simulink model "starmac_system_minimal"  (Simulink 7.1)
settings: Solver=ode45  StartTime=0.0  StopTime=30  FixedStep=.001  MaxStep=.01  RelTol=1e-4
settings Model: Creator=Administrator  LastModifiedBy=Administrator

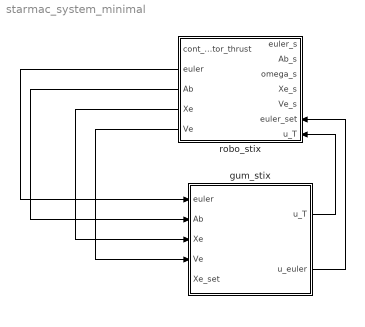
== system starmac_system_minimal ==
  gum_stix : Subsystem
  robo_stix : Subsystem  Orientation=left
  wires:
  robo_stix/2(euler) -> gum_stix/1(euler)
  robo_stix/4(Xe) -> gum_stix/3(Xe)
  robo_stix/5(Ve) -> gum_stix/4(Ve)
  gum_stix/1(u_T) -> robo_stix/7(u_T)
  gum_stix/2(u_euler) -> robo_stix/6(euler_set)
  robo_stix/3(Ab) -> gum_stix/2(Ab)

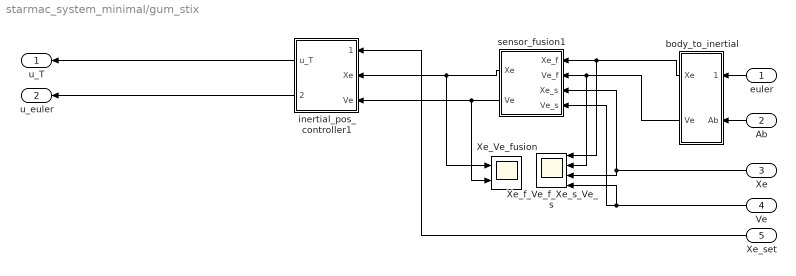
== system starmac_system_minimal/gum_stix ==
  euler : Inport  Orientation=left  PortDimensions=3  DataType=single  OutDataTypeStr=single
  Ab : Inport  Orientation=left  Port=2  PortDimensions=3  DataType=single  OutDataTypeStr=single
  Xe : Inport  Orientation=left  Port=3  PortDimensions=3  DataType=single  OutDataTypeStr=single
  Ve : Inport  Orientation=left  Port=4  PortDimensions=3  DataType=single  OutDataTypeStr=single
  Xe_set : Inport  Orientation=left  Port=5  PortDimensions=3  DataType=single  OutDataTypeStr=single
  Xe_Ve_fusion : Scope  NumInputPorts=2
      settings: YMin=-10~-5  YMax=10~5  SaveName=ScopeData2
  Xe_f_Ve_f_Xe_s_Ve_s : Scope  NumInputPorts=4
      settings: YMin=-5~-5~-5~-5  YMax=5~5~5~5  SaveName=ScopeData3
  body_to_inertial : Subsystem  Orientation=left
  inertial_pos_controller1 : Subsystem  Orientation=left
  sensor_fusion1 : Subsystem  Orientation=left
  u_T : Outport  Orientation=left  PortDimensions=1  DataType=single  OutDataTypeStr=single
  u_euler : Outport  Orientation=left  Port=2  PortDimensions=3  DataType=single  OutDataTypeStr=single
  wires:
  Xe_set/1 -> inertial_pos_controller1/1(Xe_set)
  inertial_pos_controller1/1(u_T) -> u_T/1
  inertial_pos_controller1/2(u_euler) -> u_euler/1
  euler/1 -> body_to_inertial/1(euler)
  Ab/1 -> body_to_inertial/2(Ab)
  sensor_fusion1/1(Xe) -> Xe_Ve_fusion/1, inertial_pos_controller1/2(Xe)
  sensor_fusion1/2(Ve) -> Xe_Ve_fusion/2, inertial_pos_controller1/3(Ve)
  body_to_inertial/1(Xe) -> Xe_f_Ve_f_Xe_s_Ve_s/1, sensor_fusion1/1(Xe_f)
  body_to_inertial/2(Ve) -> Xe_f_Ve_f_Xe_s_Ve_s/2, sensor_fusion1/2(Ve_f)
  Xe/1 -> Xe_f_Ve_f_Xe_s_Ve_s/3, sensor_fusion1/3(Xe_s)
  Ve/1 -> Xe_f_Ve_f_Xe_s_Ve_s/4, sensor_fusion1/4(Ve_s)

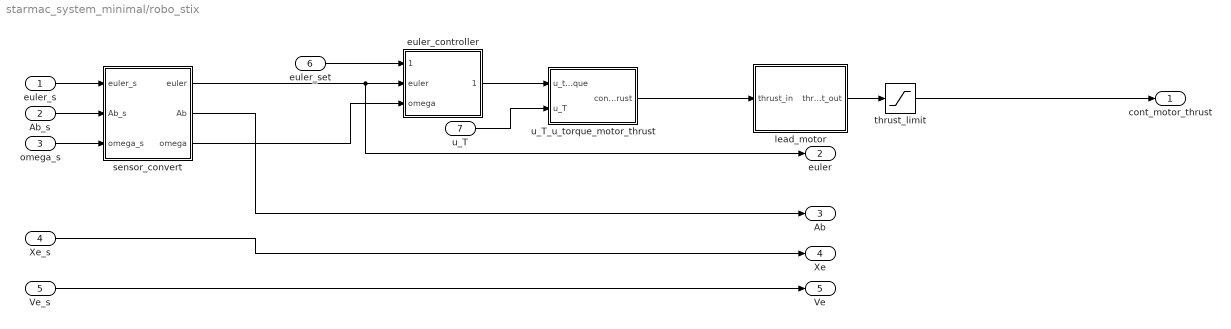
== system starmac_system_minimal/robo_stix ==
  euler_s : Inport  PortDimensions=3  DataType=single  OutDataTypeStr=single
  Ab_s : Inport  Port=2  PortDimensions=3  DataType=single  OutDataTypeStr=single
  omega_s : Inport  Port=3  PortDimensions=3  DataType=single  OutDataTypeStr=single
  Xe_s : Inport  Port=4  PortDimensions=3  DataType=single  OutDataTypeStr=single
  Ve_s : Inport  Port=5  PortDimensions=3  DataType=single  OutDataTypeStr=single
  euler_set : Inport  Port=6  PortDimensions=3  DataType=single  OutDataTypeStr=single
  u_T : Inport  Port=7  PortDimensions=1  DataType=single  OutDataTypeStr=single
  euler_controller : Subsystem  mask{K=1, K_e=7.5, K_o=.65}
      mask prompts: K "Loop Gain [K]:"; K_e "Euler Gain [K_e]:"; K_o "Omega Gain [K_o]:"
  lead_motor : Subsystem  mask{tau_motor=.10, t_s=.020}
      mask init:
      | a=1/tau_motor;
      | b=pi/t_s;
      | T=t_s;
      | num1=b*(1-exp(-b*T))+a*(b*T-1+exp(-b*T));
      | num2=-b*(1-exp(-b*T))+a*(1-exp(-b*T)-b*T*exp(-b*T));
      | den1=a*b;
      | den2=-a*b*exp(-b*T);
      | num=[num1 num2];
      | den=[den1 den2];
      | Hz=tf(num,den,T);
      | [y,t]=step(Hz);
      | k_ss=(1/y(length(y)));
      | num=k_ss*num;
      | lead_a_1=single(-den(2)/den(1))
      | lead_b_1=single(num(2)/den(1))
      | lead_b_2=single(num(1)/den(1))
      | %Hz=k_ss*Hz
      | %bode(Hz);
  sensor_convert : Subsystem  mask{a_g_s=7000, g_g_s=8500}
      mask prompts: a_g_s "AccelGainScale[a_g_s]:"; g_g_s "GyroGainScale[g_g_s]:"
  thrust_limit : Saturate  UpperLimit=10*ones(1,4)  LowerLimit=0*ones(1,4)  OutDataTypeMode=single  OutDataType=sfix(16)  OutScaling=2^0  OutDataTypeStr=single
  u_T_u_torque_motor_thrust : Subsystem  mask{dx=.3048, K_torque=.47}
      mask prompts: dx "X distance of motor from CG [dx](meters):"; K_torque "Ktorque [K_torque]:"
      mask init:
      | M=[0 -dx 0 dx;
      |    dx 0 -dx 0;
      |    -K_torque K_torque -K_torque K_torque;
      |    1 1 1 1];
      | Mi=inv(M);
  cont_motor_thrust : Outport  PortDimensions=4  DataType=single  OutDataTypeStr=single
  euler : Outport  Port=2
  Ab : Outport  Port=3
  Xe : Outport  Port=4
  Ve : Outport  Port=5
  wires:
  euler_s/1 -> sensor_convert/1(euler_s)
  Ab_s/1 -> sensor_convert/2(Ab_s)
  omega_s/1 -> sensor_convert/3(omega_s)
  sensor_convert/1(euler) -> euler/1, euler_controller/2(euler)
  euler_set/1 -> euler_controller/1(euler_set)
  sensor_convert/3(omega) -> euler_controller/3(omega)
  u_T/1 -> u_T_u_torque_motor_thrust/2(u_T)
  Xe_s/1 -> Xe/1
  Ve_s/1 -> Ve/1
  euler_controller/1(u_torque) -> u_T_u_torque_motor_thrust/1(u_torque)
  sensor_convert/2(Ab) -> Ab/1
  u_T_u_torque_motor_thrust/1(cont_motor_thrust) -> lead_motor/1(thrust_in)
  thrust_limit/1 -> cont_motor_thrust/1
  lead_motor/1(thrust_out) -> thrust_limit/1

== system starmac_system_minimal/gum_stix/body_to_inertial ==
  euler : Inport  DataType=single  OutDataTypeStr=single
  Ab : Inport  Port=2  DataType=single  OutDataTypeStr=single
  Ab_to_Ae : Stateflow chart
  inertial_vel_and pos_est : Subsystem  mask{Ts=.02}
      mask prompts: Ts "Sample Time [Ts] (seconds):"
  Xe : Outport
  Ve : Outport  Port=2
  wires:
  inertial_vel_and pos_est/2(Xb) -> Xe/1
  inertial_vel_and pos_est/1(Vb) -> Ve/1
  Ab_to_Ae/1(Ae) -> inertial_vel_and pos_est/1(Ab)
  Ab/1 -> Ab_to_Ae/2(Ab)
  euler/1 -> Ab_to_Ae/1(euler)

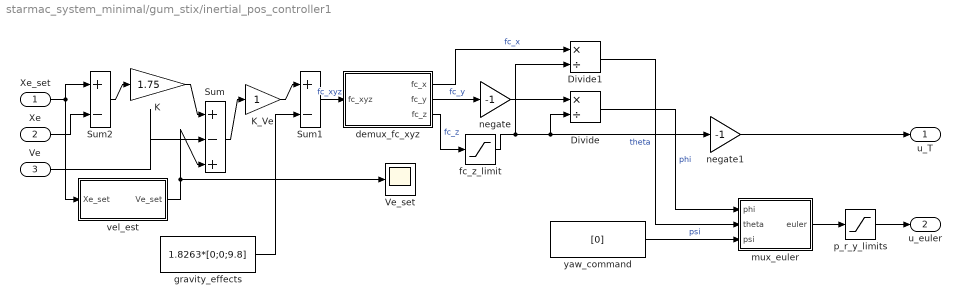
== system starmac_system_minimal/gum_stix/inertial_pos_controller1 ==
  Xe_set : Inport
  Xe : Inport  Port=2
  Ve : Inport  Port=3
  Divide : Product  Inputs=*/  OutDataTypeMode=single  OutDataType=sfix(16)  OutScaling=2^-10  OutDataTypeStr=single
  Divide1 : Product  Inputs=*/  OutDataTypeMode=single  OutDataType=sfix(16)  OutScaling=2^-10  OutDataTypeStr=single
  K : Gain  Gain=1.75  ParameterDataTypeMode=single  ParameterDataType=sfix(16)  ParameterScaling=2^0  ParamDataTypeStr=single  OutDataTypeMode=single  OutDataType=sfix(16)  OutScaling=2^0  OutDataTypeStr=single
  K_Ve : Gain  ParameterDataTypeMode=single  ParameterDataType=sfix(16)  ParameterScaling=2^0  ParamDataTypeStr=single  OutDataTypeMode=single  OutDataType=sfix(16)  OutScaling=2^0  OutDataTypeStr=single
  Sum : Sum  Inputs=|+-+  AccumDataTypeStr=single  OutDataTypeMode=single  OutDataType=sfix(16)  OutScaling=2^0  OutDataTypeStr=single
  Sum1 : Sum  Inputs=|+-  AccumDataTypeStr=single  OutDataTypeMode=single  OutDataType=sfix(16)  OutScaling=2^0  OutDataTypeStr=single
  Sum2 : Sum  Inputs=|+-  AccumDataTypeStr=single  OutDataTypeMode=single  OutDataType=sfix(16)  OutScaling=2^0  OutDataTypeStr=single
  Ve_set : Scope
      settings: SaveName=ScopeData2  Decimation=10
  demux_fc_xyz : Stateflow chart
  fc_z_limit : Saturate  UpperLimit=-(1/4)*9.81  LowerLimit=-4*9.81  OutDataTypeMode=single  OutDataType=sfix(16)  OutScaling=2^0  OutDataTypeStr=single
  gravity_effects : Constant  Value=1.8263*[0;0;9.8]  OutDataTypeMode=single  OutDataType=sfix(16)  OutScaling=2^0  OutDataTypeStr=single
  mux_euler : Stateflow chart
  negate : Gain  Gain=-1  ParameterDataTypeMode=single  ParameterDataType=sfix(16)  ParameterScaling=2^0  ParamDataTypeStr=single  OutDataTypeMode=single  OutDataType=sfix(16)  OutScaling=2^0  OutDataTypeStr=single
  negate1 : Gain  Gain=-1  ParameterDataTypeMode=single  ParameterDataType=sfix(16)  ParameterScaling=2^0  ParamDataTypeStr=single  OutDataTypeMode=single  OutDataType=sfix(16)  OutScaling=2^0  OutDataTypeStr=single
  p_r_y_limits : Saturate  UpperLimit=(pi/4)*ones(1,3)  LowerLimit=-(pi/4)*ones(1,3)  OutDataTypeMode=single  OutDataType=sfix(16)  OutScaling=2^0  OutDataTypeStr=single
  vel_est : Subsystem  mask{tau_f=.02/pi, T=.02}
      mask prompts: T "sample rate"
      mask init:
      | b=1/tau_f;
      | num1=(1-exp(-b*T));
      | num2=-num1;
      | den1=1;
      | den2=-exp(-b*T);
      | num=(1/T)*[num1 num2];
      | den=[den1 den2];
      | vel_est_a_1=single(-den(2)/den(1))
      | vel_est_b_1=single(num(2)/den(1))
      | vel_est_b_2=single(num(1)/den(1))
      | %Hz=tf(num,den,T);
      | %bode(Hz);
      | %hold on;
      | %bode(tf([1 0],[tau_f 1]));
  yaw_command : Constant  Value=[0]  OutDataTypeMode=single  OutDataType=sfix(16)  OutScaling=2^0  OutDataTypeStr=single
  u_T : Outport  DataType=single  OutDataTypeStr=single
  u_euler : Outport  Port=2  PortDimensions=[3]  DataType=single  OutDataTypeStr=single
  wires:
  vel_est/1(Ve_set) -> Ve_set/1, Sum/3
  Ve/1 -> Sum/2
  K_Ve/1 -> Sum1/1
  demux_fc_xyz/2(fc_y) -> negate/1  "fc_y"
  K/1 -> Sum/1
  Sum2/1 -> K/1
  Xe/1 -> Sum2/2
  Sum/1 -> K_Ve/1
  gravity_effects/1 -> Sum1/2
  Sum1/1 -> demux_fc_xyz/1(fc_xyz)  "fc_xyz"
  mux_euler/1(euler) -> p_r_y_limits/1
  demux_fc_xyz/3(fc_z) -> fc_z_limit/1  "fc_z"
  yaw_command/1 -> mux_euler/3(psi)  "psi"
  negate/1 -> Divide/1
  Divide/1 -> mux_euler/1(phi)  "phi"
  demux_fc_xyz/1(fc_x) -> Divide1/1  "fc_x"
  Divide1/1 -> mux_euler/2(theta)  "theta"
  p_r_y_limits/1 -> u_euler/1
  negate1/1 -> u_T/1
  Xe_set/1 -> vel_est/1(Xe_set), Sum2/1
  fc_z_limit/1 -> negate1/1, Divide/2, Divide1/2

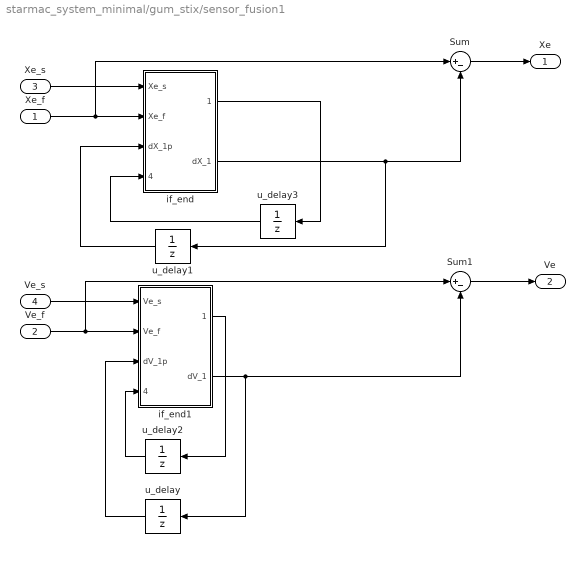
== system starmac_system_minimal/gum_stix/sensor_fusion1 ==
  Xe_f : Inport
  Ve_f : Inport  Port=2
  Xe_s : Inport  Port=3
  Ve_s : Inport  Port=4
  Sum : Sum  Inputs=|+-  OutDataTypeMode=single  OutDataType=sfix(16)  OutScaling=2^0  OutDataTypeStr=single
  Sum1 : Sum  Inputs=|+-  OutDataTypeMode=single  OutDataType=sfix(16)  OutScaling=2^0  OutDataTypeStr=single
  if_end : Subsystem
  if_end1 : Subsystem
  u_delay{,1..3} (4 alike) : UnitDelay  Orientation=left  SampleTime=-1
  Xe : Outport
  Ve : Outport  Port=2
  wires:
  Sum1/1 -> Ve/1
  Sum/1 -> Xe/1
  if_end/1(Xe_sh_1) -> u_delay3/1
  if_end1/1(Ve_sh_1) -> u_delay2/1
  if_end1/2(dV_1) -> Sum1/2, u_delay/1
  if_end/2(dX_1) -> Sum/2, u_delay1/1
  u_delay2/1 -> if_end1/4(Ve_sh_1p)
  u_delay/1 -> if_end1/3(dV_1p)
  Ve_s/1 -> if_end1/1(Ve_s)
  Ve_f/1 -> Sum1/1, if_end1/2(Ve_f)
  u_delay3/1 -> if_end/4(Xe_sh_1p)
  Xe_s/1 -> if_end/1(Xe_s)
  u_delay1/1 -> if_end/3(dX_1p)
  Xe_f/1 -> Sum/1, if_end/2(Xe_f)

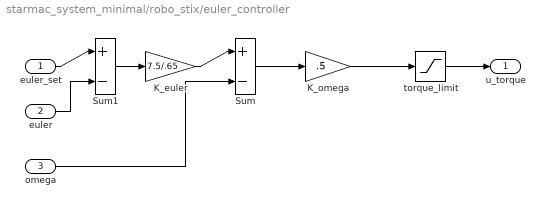
== system starmac_system_minimal/robo_stix/euler_controller ==
  euler_set : Inport
  euler : Inport  Port=2
  omega : Inport  Port=3
  K_euler : Gain  Gain=7.5/.65  ParameterDataTypeMode=single  ParameterDataType=sfix(16)  ParameterScaling=2^0  ParamDataTypeStr=single  OutDataTypeMode=single  OutDataType=sfix(16)  OutScaling=2^0  OutDataTypeStr=single
  K_omega : Gain  Gain=.5  ParameterDataTypeMode=single  ParameterDataType=sfix(16)  ParameterScaling=2^0  ParamDataTypeStr=single  OutDataTypeMode=single  OutDataType=sfix(16)  OutScaling=2^0  OutDataTypeStr=single
  Sum : Sum  Inputs=|+-  AccumDataTypeStr=single  OutDataTypeMode=single  OutDataType=sfix(16)  OutScaling=2^0  OutDataTypeStr=single
  Sum1 : Sum  Inputs=|+-  AccumDataTypeStr=single  OutDataTypeMode=single  OutDataType=sfix(16)  OutScaling=2^0  OutDataTypeStr=single
  torque_limit : Saturate  UpperLimit=9.8*.3048*ones(3,1)  LowerLimit=-9.8*.3048*ones(3,1)  OutDataTypeMode=single  OutDataType=sfix(16)  OutScaling=2^0  OutDataTypeStr=single
  u_torque : Outport
  wires:
  Sum/1 -> K_omega/1
  euler_set/1 -> Sum1/1
  Sum1/1 -> K_euler/1
  euler/1 -> Sum1/2
  K_euler/1 -> Sum/1
  torque_limit/1 -> u_torque/1
  K_omega/1 -> torque_limit/1
  omega/1 -> Sum/2

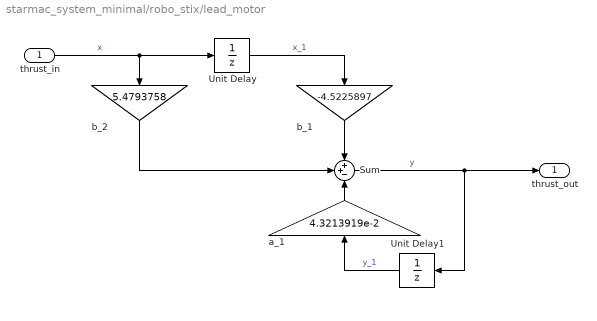
== system starmac_system_minimal/robo_stix/lead_motor ==
  thrust_in : Inport  DataType=single  OutDataTypeStr=single
  Sum : Sum  Inputs=++-  AccumDataTypeStr=single  OutDataTypeMode=single  OutDataType=sfix(16)  OutScaling=2^0  OutDataTypeStr=single
  Unit Delay : UnitDelay  SampleTime=-1
  Unit Delay1 : UnitDelay  Orientation=left  SampleTime=-1
  a_1 : Gain  Orientation=up  Gain=4.3213919e-2  ParameterDataTypeMode=single  ParameterDataType=sfix(16)  ParameterScaling=2^0  ParamDataTypeStr=single  OutDataTypeMode=single  OutDataType=sfix(16)  OutScaling=2^0  OutDataTypeStr=single
  b_1 : Gain  Orientation=down  Gain=-4.5225897  ParameterDataTypeMode=single  ParameterDataType=sfix(16)  ParameterScaling=2^0  ParamDataTypeStr=single  OutDataTypeMode=single  OutDataType=sfix(16)  OutScaling=2^0  OutDataTypeStr=single
  b_2 : Gain  Orientation=down  Gain=5.4793758  ParameterDataTypeMode=single  ParameterDataType=sfix(16)  ParameterScaling=2^0  ParamDataTypeStr=single  OutDataTypeMode=single  OutDataType=sfix(16)  OutScaling=2^0  OutDataTypeStr=single
  thrust_out : Outport  DataType=single  OutDataTypeStr=single
  wires:
  thrust_in/1 -> Unit Delay/1, b_2/1  "x"
  Unit Delay/1 -> b_1/1  "x_1"
  b_1/1 -> Sum/1
  b_2/1 -> Sum/2
  Sum/1 -> thrust_out/1, Unit Delay1/1  "y"
  a_1/1 -> Sum/3
  Unit Delay1/1 -> a_1/1  "y_1"

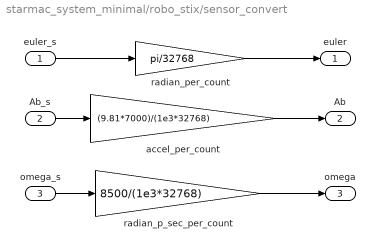
== system starmac_system_minimal/robo_stix/sensor_convert ==
  euler_s : Inport
  Ab_s : Inport  Port=2
  omega_s : Inport  Port=3
  accel_per_count : Gain  Gain=(9.81*7000)/(1e3*32768)  ParameterDataTypeMode=single  ParameterDataType=sfix(16)  ParameterScaling=2^0  ParamDataTypeStr=single  OutDataTypeMode=single  OutDataType=sfix(16)  OutScaling=2^0  OutDataTypeStr=single
  radian_p_sec_per_count : Gain  Gain=8500/(1e3*32768)  ParameterDataTypeMode=single  ParameterDataType=sfix(16)  ParameterScaling=2^0  ParamDataTypeStr=single  OutDataTypeMode=single  OutDataType=sfix(16)  OutScaling=2^0  OutDataTypeStr=single
  radian_per_count : Gain  Gain=pi/32768  ParameterDataTypeMode=single  ParameterDataType=sfix(16)  ParameterScaling=2^0  ParamDataTypeStr=single  OutDataTypeMode=single  OutDataType=sfix(16)  OutScaling=2^0  OutDataTypeStr=single
  euler : Outport
  Ab : Outport  Port=2
  omega : Outport  Port=3
  wires:
  euler_s/1 -> radian_per_count/1
  radian_per_count/1 -> euler/1
  Ab_s/1 -> accel_per_count/1
  accel_per_count/1 -> Ab/1
  omega_s/1 -> radian_p_sec_per_count/1
  radian_p_sec_per_count/1 -> omega/1

== system starmac_system_minimal/robo_stix/u_T_u_torque_motor_thrust ==
  u_torque : Inport  DataType=single  OutDataTypeStr=single
  u_T : Inport  Port=2  DataType=single  OutDataTypeStr=single
  Mi : Gain  Gain=[0,1.6404,-.5319,.25;-1.6404,0,.5319,.25;0,-1.6404,-.5319,.25;1.6404,0,.5319,.25]  Multiplication=Matrix(K*u)  ParameterDataTypeMode=single  ParameterDataType=sfix(16)  ParameterScaling=2^0  ParamDataTypeStr=single  OutDataTypeMode=single  OutDataType=sfix(16)  OutScaling=2^0  OutDataTypeStr=single
  u_torque_u_T_mux : Stateflow chart
  cont_motor_thrust : Outport  DataType=single  OutDataTypeStr=single
  wires:
  u_torque/1 -> u_torque_u_T_mux/1(u_torque)
  u_T/1 -> u_torque_u_T_mux/2(u_T)
  Mi/1 -> cont_motor_thrust/1
  u_torque_u_T_mux/1(u_torque_u_T) -> Mi/1

== system starmac_system_minimal/gum_stix/body_to_inertial/inertial_vel_and pos_est ==
  Ab : Inport  PortDimensions=[3]  DataType=single  OutDataTypeStr=single
  DT_integrator : Subsystem
  DT_integrator1 : Subsystem
  Vb : Outport
  Xb : Outport  Port=2
  wires:
  DT_integrator/1(Vb) -> DT_integrator1/1(Vb), Vb/1
  Ab/1 -> DT_integrator/1(Ab)
  DT_integrator1/1(Xb) -> Xb/1

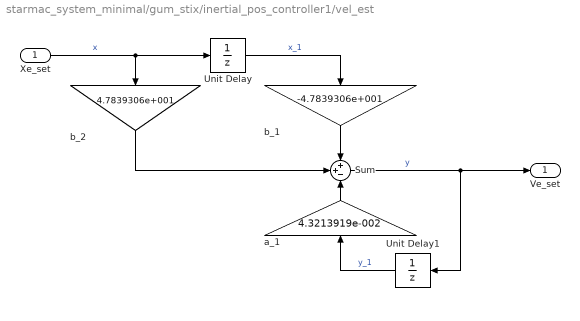
== system starmac_system_minimal/gum_stix/inertial_pos_controller1/vel_est ==
  Xe_set : Inport  DataType=single  OutDataTypeStr=single
  Sum : Sum  Inputs=++-  AccumDataTypeStr=single  OutDataTypeMode=single  OutDataType=sfix(16)  OutScaling=2^0  OutDataTypeStr=single
  Unit Delay : UnitDelay  SampleTime=-1
  Unit Delay1 : UnitDelay  Orientation=left  SampleTime=-1
  a_1 : Gain  Orientation=up  Gain=4.3213919e-002  ParameterDataTypeMode=single  ParameterDataType=sfix(16)  ParameterScaling=2^0  ParamDataTypeStr=single  OutDataTypeMode=single  OutDataType=sfix(16)  OutScaling=2^0  OutDataTypeStr=single
  b_1 : Gain  Orientation=down  Gain=-4.7839306e+001  ParameterDataTypeMode=single  ParameterDataType=sfix(16)  ParameterScaling=2^0  ParamDataTypeStr=single  OutDataTypeMode=single  OutDataType=sfix(16)  OutScaling=2^0  OutDataTypeStr=single
  b_2 : Gain  Orientation=down  Gain=4.7839306e+001  ParameterDataTypeMode=single  ParameterDataType=sfix(16)  ParameterScaling=2^0  ParamDataTypeStr=single  OutDataTypeMode=single  OutDataType=sfix(16)  OutScaling=2^0  OutDataTypeStr=single
  Ve_set : Outport
  wires:
  Unit Delay1/1 -> a_1/1  "y_1"
  a_1/1 -> Sum/3
  Sum/1 -> Ve_set/1, Unit Delay1/1  "y"
  b_2/1 -> Sum/2
  b_1/1 -> Sum/1
  Unit Delay/1 -> b_1/1  "x_1"
  Xe_set/1 -> b_2/1, Unit Delay/1  "x"

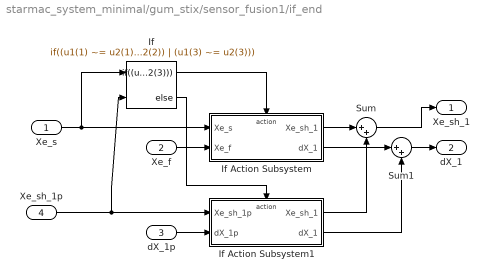
== system starmac_system_minimal/gum_stix/sensor_fusion1/if_end ==
  Xe_s : Inport
  Xe_f : Inport  Port=2
  dX_1p : Inport  Port=3
  Xe_sh_1p : Inport  Port=4
  If : If  NumInputs=2  IfExpression=(u1(1) ~= u2(1)) | (u1(2) ~= u2(2)) | (u1(3) ~= u2(3))
  If Action Subsystem : Subsystem  TreatAsAtomicUnit=on
  If Action Subsystem1 : Subsystem  TreatAsAtomicUnit=on
  Sum : Sum  Inputs=|++  OutDataTypeMode=single  OutDataType=sfix(16)  OutScaling=2^0  OutDataTypeStr=single
  Sum1 : Sum  Inputs=|++  OutDataTypeMode=single  OutDataType=sfix(16)  OutScaling=2^0  OutDataTypeStr=single
  Xe_sh_1 : Outport
  dX_1 : Outport  Port=2
  wires:
  dX_1p/1 -> If Action Subsystem1/2(dX_1p)
  Sum1/1 -> dX_1/1
  Xe_f/1 -> If Action Subsystem/2(Xe_f)
  Sum/1 -> Xe_sh_1/1
  If Action Subsystem1/2(dX_1) -> Sum1/2
  If Action Subsystem1/1(Xe_sh_1) -> Sum/2
  If Action Subsystem/2(dX_1) -> Sum1/1
  If Action Subsystem/1(Xe_sh_1) -> Sum/1
  Xe_sh_1p/1 -> If Action Subsystem1/1(Xe_sh_1p), If/2
  Xe_s/1 -> If/1, If Action Subsystem/1(Xe_s)
  If/2 -> If Action Subsystem1/Action
  If/1 -> If Action Subsystem/Action

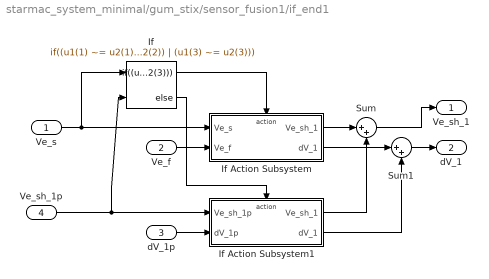
== system starmac_system_minimal/gum_stix/sensor_fusion1/if_end1 ==
  Ve_s : Inport
  Ve_f : Inport  Port=2
  dV_1p : Inport  Port=3
  Ve_sh_1p : Inport  Port=4
  If : If  NumInputs=2  IfExpression=(u1(1) ~= u2(1)) | (u1(2) ~= u2(2)) | (u1(3) ~= u2(3))
  If Action Subsystem : Subsystem  TreatAsAtomicUnit=on
  If Action Subsystem1 : Subsystem  TreatAsAtomicUnit=on
  Sum : Sum  Inputs=|++  OutDataTypeMode=single  OutDataType=sfix(16)  OutScaling=2^0  OutDataTypeStr=single
  Sum1 : Sum  Inputs=|++  OutDataTypeMode=single  OutDataType=sfix(16)  OutScaling=2^0  OutDataTypeStr=single
  Ve_sh_1 : Outport
  dV_1 : Outport  Port=2
  wires:
  If/1 -> If Action Subsystem/Action
  If/2 -> If Action Subsystem1/Action
  Ve_s/1 -> If Action Subsystem/1(Ve_s), If/1
  Ve_sh_1p/1 -> If/2, If Action Subsystem1/1(Ve_sh_1p)
  If Action Subsystem/1(Ve_sh_1) -> Sum/1
  If Action Subsystem/2(dV_1) -> Sum1/1
  If Action Subsystem1/1(Ve_sh_1) -> Sum/2
  If Action Subsystem1/2(dV_1) -> Sum1/2
  Sum/1 -> Ve_sh_1/1
  Ve_f/1 -> If Action Subsystem/2(Ve_f)
  Sum1/1 -> dV_1/1
  dV_1p/1 -> If Action Subsystem1/2(dV_1p)

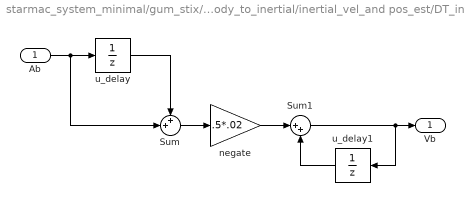
== system starmac_system_minimal/gum_stix/body_to_inertial/inertial_vel_and pos_est/DT_integrator ==
  Ab : Inport  DataType=single  OutDataTypeStr=single
  Sum : Sum  Inputs=++|  AccumDataTypeStr=single  OutDataTypeMode=single  OutDataType=sfix(16)  OutScaling=2^0  OutDataTypeStr=single
  Sum1 : Sum  Inputs=|++  AccumDataTypeStr=single  OutDataTypeMode=single  OutDataType=sfix(16)  OutScaling=2^0  OutDataTypeStr=single
  negate : Gain  Gain=.5*.02  ParameterDataTypeMode=single  ParameterDataType=sfix(16)  ParameterScaling=2^0  ParamDataTypeStr=single  OutDataTypeMode=single  OutDataType=sfix(16)  OutScaling=2^0  OutDataTypeStr=single
  u_delay : UnitDelay  SampleTime=-1
  u_delay1 : UnitDelay  Orientation=left  SampleTime=-1
  Vb : Outport  DataType=single  OutDataTypeStr=single
  wires:
  u_delay1/1 -> Sum1/2
  Sum1/1 -> Vb/1, u_delay1/1
  negate/1 -> Sum1/1
  Sum/1 -> negate/1
  u_delay/1 -> Sum/1
  Ab/1 -> Sum/2, u_delay/1

== system starmac_system_minimal/gum_stix/body_to_inertial/inertial_vel_and pos_est/DT_integrator1 ==
  Vb : Inport  DataType=single  OutDataTypeStr=single
  Sum : Sum  Inputs=++|  AccumDataTypeStr=single  OutDataTypeMode=single  OutDataType=sfix(16)  OutScaling=2^0  OutDataTypeStr=single
  Sum1 : Sum  Inputs=|++  AccumDataTypeStr=single  OutDataTypeMode=single  OutDataType=sfix(16)  OutScaling=2^0  OutDataTypeStr=single
  negate : Gain  Gain=.5*.02  ParameterDataTypeMode=single  ParameterDataType=sfix(16)  ParameterScaling=2^0  ParamDataTypeStr=single  OutDataTypeMode=single  OutDataType=sfix(16)  OutScaling=2^0  OutDataTypeStr=single
  u_delay : UnitDelay  SampleTime=-1
  u_delay1 : UnitDelay  Orientation=left  SampleTime=-1
  Xb : Outport  PortDimensions=[3]  DataType=single  OutDataTypeStr=single
  wires:
  Vb/1 -> u_delay/1, Sum/2
  u_delay/1 -> Sum/1
  Sum/1 -> negate/1
  negate/1 -> Sum1/1
  Sum1/1 -> u_delay1/1, Xb/1
  u_delay1/1 -> Sum1/2

== system starmac_system_minimal/gum_stix/sensor_fusion1/if_end/If Action Subsystem ==
  Xe_s : Inport  OutDataType=sfix(16)  OutScaling=2^0
  Xe_f : Inport  Port=2  OutDataType=sfix(16)  OutScaling=2^0
  Action Port : ActionPort  InitializeStates=reset  ActionType=then
  Sum : Sum  Inputs=-+|  OutDataTypeMode=single  OutDataType=sfix(16)  OutScaling=2^0  OutDataTypeStr=single
  Xe_sh_1 : Outport  OutDataType=sfix(16)  OutScaling=2^0  OutputWhenDisabled=reset  InitialOutput=zeros(1,3,'single')
  dX_1 : Outport  Port=2  OutDataType=sfix(16)  OutScaling=2^0  OutputWhenDisabled=reset  InitialOutput=zeros(1,3,'single')
  wires:
  Sum/1 -> dX_1/1
  Xe_f/1 -> Sum/2
  Xe_s/1 -> Sum/1, Xe_sh_1/1

== system starmac_system_minimal/gum_stix/sensor_fusion1/if_end/If Action Subsystem1 ==
  Xe_sh_1p : Inport  OutDataType=sfix(16)  OutScaling=2^0
  dX_1p : Inport  Port=2  OutDataType=sfix(16)  OutScaling=2^0
  Action Port : ActionPort  InitializeStates=reset  ActionType=else
  Xe_sh_1 : Outport  DataType=single  OutDataType=sfix(16)  OutScaling=2^0  OutDataTypeStr=single  OutputWhenDisabled=reset  InitialOutput=zeros(1,3,'single')
  dX_1 : Outport  Port=2  DataType=single  OutDataType=sfix(16)  OutScaling=2^0  OutDataTypeStr=single  OutputWhenDisabled=reset  InitialOutput=zeros(1,3,'single')
  wires:
  Xe_sh_1p/1 -> Xe_sh_1/1
  dX_1p/1 -> dX_1/1

== system starmac_system_minimal/gum_stix/sensor_fusion1/if_end1/If Action Subsystem ==
  Ve_s : Inport  OutDataType=sfix(16)  OutScaling=2^0
  Ve_f : Inport  Port=2  OutDataType=sfix(16)  OutScaling=2^0
  Action Port : ActionPort  InitializeStates=reset  ActionType=then
  Sum : Sum  Inputs=-+|  OutDataTypeMode=single  OutDataType=sfix(16)  OutScaling=2^0  OutDataTypeStr=single
  Ve_sh_1 : Outport  OutDataType=sfix(16)  OutScaling=2^0  OutputWhenDisabled=reset  InitialOutput=zeros(1,3,'single')
  dV_1 : Outport  Port=2  OutDataType=sfix(16)  OutScaling=2^0  OutputWhenDisabled=reset  InitialOutput=zeros(1,3,'single')
  wires:
  Ve_s/1 -> Ve_sh_1/1, Sum/1
  Ve_f/1 -> Sum/2
  Sum/1 -> dV_1/1

== system starmac_system_minimal/gum_stix/sensor_fusion1/if_end1/If Action Subsystem1 ==
  Ve_sh_1p : Inport  OutDataType=sfix(16)  OutScaling=2^0
  dV_1p : Inport  Port=2  OutDataType=sfix(16)  OutScaling=2^0
  Action Port : ActionPort  InitializeStates=reset  ActionType=else
  Ve_sh_1 : Outport  DataType=single  OutDataType=sfix(16)  OutScaling=2^0  OutDataTypeStr=single  OutputWhenDisabled=reset  InitialOutput=zeros(1,3,'single')
  dV_1 : Outport  Port=2  DataType=single  OutDataType=sfix(16)  OutScaling=2^0  OutDataTypeStr=single  OutputWhenDisabled=reset  InitialOutput=zeros(1,3,'single')
  wires:
  dV_1p/1 -> dV_1/1
  Ve_sh_1p/1 -> Ve_sh_1/1

== matlab function gum_stix/inertial_pos_controller1/mux_euler ==
  data: phi input single size=[1]; euler output single size=[3]; theta input single size=[1]; psi input single size=[1]
function euler = fcn(phi, theta, psi)
% This block supports the Embedded MATLAB subset.
% See the help menu for details. 
euler=[phi;theta;psi];

== matlab function gum_stix/inertial_pos_controller1/demux_fc_xyz ==
  data: fc_xyz input single size=[3]; fc_x output single size=[1]; fc_y output single size=[1]; fc_z output single size=[1]
function [fc_x,fc_y, fc_z] = fcn(fc_xyz)
% This block supports the Embedded MATLAB subset.
% See the help menu for details. 
fc_x=fc_xyz(1);
fc_y=fc_xyz(2);
fc_z=fc_xyz(3);

== matlab function robo_stix/u_T_u_torque_motor_thrust/u_torque_u_T_mux ==
  data: u_torque input single size=[3]; u_torque_u_T output single size=[4]; u_T input single size=[1]
function u_torque_u_T = fcn(u_torque, u_T)
% This block supports the Embedded MATLAB subset.
% See the help menu for details. 
u_torque_u_T = [u_torque; u_T];

== matlab function gum_stix/body_to_inertial/Ab_to_Ae ==
  data: euler input single size=[3]; Ae output single size=[3]; Ab input single size=[3]
function Ae = fcn(euler, Ab)
% This block supports the Embedded MATLAB subset.
% See the help menu for details. 
phi=euler(1);
theta=euler(2);
psi=euler(3);
c_phi=cos(phi);
c_theta=cos(theta);
c_psi=cos(psi);
s_phi=sin(phi);
s_theta=sin(theta);
s_psi=sin(psi);
R=[c_theta*c_psi, c_theta*s_psi, -s_theta;s_phi*s_theta*c_psi-c_phi*s_psi, s_phi*s_theta*s_psi+c_phi*c_psi, c_theta*s_phi;c_phi*s_theta*c_psi+s_phi*s_psi, c_phi*s_theta*s_psi-s_phi*c_psi, c_theta*c_phi];
%R=single(zeros(3,3));
%R(1,1)=c_theta*c_psi;
%R(1,2)=c_theta*s_psi;
%R(1,3)=-s_theta;
%R(2,1)=s_phi*s_theta*c_psi - c_phi*s_psi;
%R(2,2)=s_phi*s_theta*s_psi + c_phi*c_psi;
%R(2,3)=c_theta*s_phi;
%R(3,1)=c_phi*s_theta*c_psi + s_phi*s_psi;
%R(3,2)=c_phi*s_theta*s_psi - s_phi*c_psi;
%R(3,3)=c_theta*c_phi;
Ae= transpose(R) * Ab;
%Ae= single(Aed);
